simulink model "B_LPV_Sim"  (R2020a)
settings: Solver=VariableStepAuto  StartTime=0.0  StopTime=10.0  FixedStep=5e-3  RelTol=1e-3
values from neighbouring files (symbols this model uses):
  b_LPV = b(:)    [B_LPV.m]    (also in B_LPV2.m)
  k = 10    [B_LPV.m]    (also in B_LPV2.m)
  K_LPV = K(:)    [B_LPV.m]    (also in B_LPV2.m)
  x0 = 2    [B_LPV.m]    (also in B_LPV2.m)
settings Model: Creator=FawaD KhaN  LastModifiedBy=FawaD KhaN
settings DebuggingCC: StringTruncationChecking=none

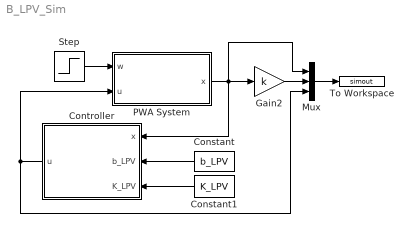
== system B_LPV_Sim ==
  Constant : Constant  Value=b_LPV
  Constant1 : Constant  Value=K_LPV
  Controller : MATLAB Function  TreatAsAtomicUnit=on
  Gain2 : Gain  Gain=k
  Mux : Mux  Inputs=3
  PWA System : Subsystem
  Step : Step  Time=0  SampleTime=0
  To Workspace : ToWorkspace  VariableName=simout  SaveFormat=Timeseries  SampleTime=-1
  wires:
  PWA System/1(x) -> Controller/1(x), Mux/1, Gain2/1
  Step/1 -> PWA System/1(w)
  Controller/1(u) -> Mux/3, PWA System/2(u)
  Gain2/1 -> Mux/2
  Mux/1 -> To Workspace/1
  Constant/1 -> Controller/2(b_LPV)
  Constant1/1 -> Controller/3(K_LPV)

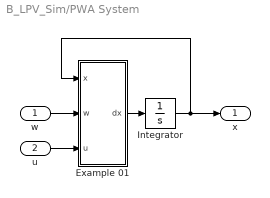
== system B_LPV_Sim/PWA System ==
  w : Inport
  u : Inport  Port=2
  Example 01 : MATLAB Function  TreatAsAtomicUnit=on
  Integrator : Integrator  InitialCondition=x0
  x : Outport
  wires:
  u/1 -> Example 01/3(u)
  Example 01/1(dx) -> Integrator/1
  Integrator/1 -> Example 01/1(x), x/1
  w/1 -> Example 01/2(w)

== matlab function B_LPV_Sim/PWA System/Example 01 ==
  data: x input; w input; u input; dx output
function dx = fcn(x,w,u)

dx = -5*x*(1+(sin(x))^2) + w + u;

end

== matlab function B_LPV_Sim/Controller ==
  data: x input; b_LPV input; u output; K_LPV input
function u  = fcn(x,b_LPV,K_LPV)

K = interp1(b_LPV,K_LPV,x);

u = K*x;

end
